simulink model "robot2bactudo"  (R2021a)
settings: Solver=FixedStepAuto  StartTime=0.0  StopTime=60  FixedStep=0.01  RelTol=1e-3
values from neighbouring files (symbols this model uses):
  g = 9.81    [robot2bac.m]
  l1 = 1    [robot2bac.m]
  l2 = 1    [robot2bac.m]
  m1 = 1    [robot2bac.m]
  m2 = 1    [robot2bac.m]
  teta2_init = 0.001    [robot2bac.m]
settings Model: Creator=Admin  LastModifiedBy=Admin

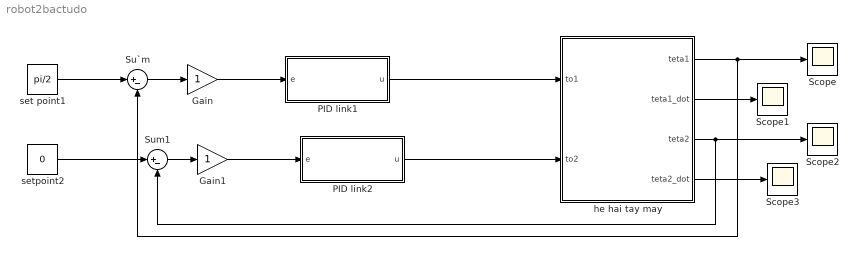
== system robot2bactudo ==
  Gain : Gain
  Gain1 : Gain
  PID link1 : Subsystem  mask{Kp=200, Ki=30, Kd=200}
  PID link2 : Subsystem  mask{Kp=250, Ki=500, Kd=200}
  Scope{,1..3} (4 alike) : Scope
  Su`m : Sum  Inputs=|+-
  Sum1 : Sum  Inputs=|+-
  he hai tay may : Subsystem
  set point1 : Constant  Value=pi/2
  setpoint2 : Constant  Value=0
  wires:
  he hai tay may/1(teta1) -> Su`m/2, Scope/1
  he hai tay may/2(teta1_dot) -> Scope1/1
  he hai tay may/3(teta2) -> Sum1/2, Scope2/1
  he hai tay may/4(teta2_dot) -> Scope3/1
  set point1/1 -> Su`m/1
  setpoint2/1 -> Sum1/1
  Su`m/1 -> Gain/1
  Sum1/1 -> Gain1/1
  Gain/1 -> PID link1/1(e)
  Gain1/1 -> PID link2/1(e)
  PID link2/1(u) -> he hai tay may/2(to2)
  PID link1/1(u) -> he hai tay may/1(to1)

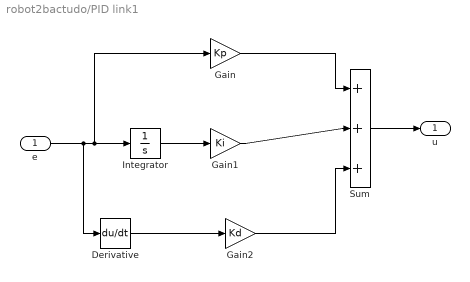
== system robot2bactudo/PID link1 ==
  e : Inport
  Derivative : Derivative
  Gain : Gain  Gain=Kp
  Gain1 : Gain  Gain=Ki
  Gain2 : Gain  Gain=Kd
  Integrator : Integrator
  Sum : Sum  Inputs=|+++
  u : Outport
  wires:
  Derivative/1 -> Gain2/1
  Integrator/1 -> Gain1/1
  e/1 -> Derivative/1, Gain/1, Integrator/1
  Gain1/1 -> Sum/2
  Gain/1 -> Sum/1
  Gain2/1 -> Sum/3
  Sum/1 -> u/1

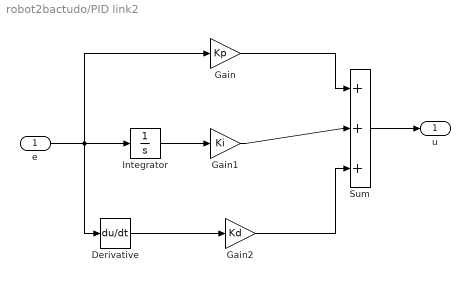
== system robot2bactudo/PID link2 ==
  e : Inport
  Derivative : Derivative
  Gain : Gain  Gain=Kp
  Gain1 : Gain  Gain=Ki
  Gain2 : Gain  Gain=Kd
  Integrator : Integrator
  Sum : Sum  Inputs=|+++
  u : Outport
  wires:
  Derivative/1 -> Gain2/1
  Integrator/1 -> Gain1/1
  Gain1/1 -> Sum/2
  Gain/1 -> Sum/1
  Gain2/1 -> Sum/3
  Sum/1 -> u/1
  e/1 -> Derivative/1, Gain/1, Integrator/1

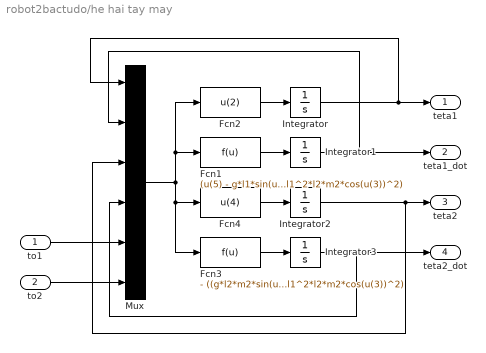
== system robot2bactudo/he hai tay may ==
  to1 : Inport
  to2 : Inport  Port=2
  Fcn1 : Fcn  Expr=(u(5) - g*l1*sin(u(1))*(m1 + m2) - g*l2*m2*sin(u(1) + u(3)) + l1*l2*m2*sin(u(3))*(u(4)^2 + 2*u(2)*u(4)))/(l1^2*m1 + l1^2*m2 - l1^2*m2*cos(u(3))^2) + ((l2 + l1*cos(u(3)))*(g*l2*m2*sin(u(1) + u(3)) - u(6) + l1*l2*m2*u(2)*u(4)*sin(u(3))))/(l1^2*l2*m1 + l1^2*l2*m2 - l1^2*l2*m2*cos(u(3))^2)
  Fcn2 : Fcn  Expr=u(2)
  Fcn3 : Fcn  Expr=- ((g*l2*m2*sin(u(1) + u(3)) - u(6) + l1*l2*m2*u(2)*u(4)*sin(u(3)))*(l1^2*m1 + l1^2*m2 + l2^2*m2 + 2*l1*l2*m2*cos(u(3))))/(- l1^2*l2^2*m2^2*cos(u(3))^2 + l1^2*l2^2*m2^2 + m1*l1^2*l2^2*m2) - ((l2 + l1*cos(u(3)))*(u(5) - g*l1*sin(u(1))*(m1 + m2) - g*l2*m2*sin(u(1) + u(3)) + l1*l2*m2*sin(u(3))*(u(4)^2 + 2*u(2)*u(4))))/(l1^2*l2*m1 + l1^2*l2*m2 - l1^2*l2*m2*cos(u(3))^2)
  Fcn4 : Fcn  Expr=u(4)
  Integrator : Integrator
  Integrator1 : Integrator
  Integrator2 : Integrator  InitialCondition=teta2_init
  Integrator3 : Integrator
  Mux : Mux  Inputs=6
  teta1 : Outport
  teta1_dot : Outport  Port=2
  teta2 : Outport  Port=3
  teta2_dot : Outport  Port=4
  wires:
  Fcn3/1 -> Integrator3/1
  Integrator1/1 -> Mux/2, teta1_dot/1
  Fcn4/1 -> Integrator2/1
  Fcn2/1 -> Integrator/1
  Integrator3/1 -> Mux/4, teta2_dot/1
  Integrator/1 -> teta1/1, Mux/1
  to2/1 -> Mux/6
  Fcn1/1 -> Integrator1/1
  Mux/1 -> Fcn4/1, Fcn3/1, Fcn2/1, Fcn1/1
  to1/1 -> Mux/5
  Integrator2/1 -> Mux/3, teta2/1
